simulink model "M10B39_es_V1"  (R2024b)
settings: Solver=ode23tb  StartTime=0.0  StopTime=20  FixedStep=0.001  RelTol=1e-3  EnableMultiTasking=on
InitFcn:
  | initAll;
values from neighbouring files (symbols this model uses):
  acom = 100    [initAll_V1.m]    (also in initAll_V2.m; initAll_V3.m; parameterinit.mat)
  AVm0 = [4.26082678503 4.656135219]    [parameterinit.mat]
  bcom = 50    [initAll_V1.m]    (also in initAll_V2.m; initAll_V3.m; parameterinit.mat)
  commun = 0*commun    [initAll_V1.m]    (also in initAll_V2.m; initAll_V3.m; parameterinit.mat = [0  0  0; 0  0  0; 0  0  0; 0  0  0])
  DataDelay = 0.0*DataDelay    [initAll_V1.m]    (also in initAll_V2.m; initAll_V3.m; parameterinit.mat = [0  0  0; 0  0  0; 0  0  0; 0  0  0])
  ESinit =     [parameterinit.mat]
  fB = 50    [initAll.m]    (also in initAll_V1.m; initAll_V2.m; initAll_V3.m; parameterinit.mat)
  Geninit = Generator_init(opdata,SynMach_in_gidx)    [initAll.m]    (also in initAll_V1.m; initAll_V2.m; initAll_V3.m = Generator_init(opdata_all,SynMach_in_gidx1); parameterinit.mat = )
  lam = 100    [initAll_V1.m]    (also in initAll_V2.m; initAll_V3.m; parameterinit.mat)
  SgridB = 100    [initAll.m]    (also in initAll_V1.m; initAll_V2.m; initAll_V3.m; parameterinit.mat)
  wB = 2*pi*fB    (= 314.159265359)    [initAll.m]    (also in initAll_V1.m; initAll_V2.m; initAll_V3.m; parameterinit.mat)
  Windinit =     [parameterinit.mat]
  YY_load = [3.65450097002 -2.05705688056 0 0 0 0 0 0 0 0 0 0 ... (1521 elements, 39x39)]    [parameterinit.mat]    (also in powerflowcaculate.m = full(YY))
undefined symbols (not defined in the file or in its folder): c1, c2, c3, c4, c5, c6, cp_nom, lambda_nom, P_wind_base, Pelec_base, Pnom
libraries: spsBistableLib x12, simulink_extras x4, slpidlib x1, simulink x1
(part 3 of 7)

== system M10B39_es_V1/Genrators/W_ES ==
  Gain1 : Gain  Gain=commun(4,1)
  Gain10 : Gain  Gain=commun(3,1)
  Gain11 : Gain  Gain=commun(1,2)
  Gain12 : Gain  Gain=commun(2,1)
  Gain13 : Gain  Gain=commun(8,2)
  Gain2 : Gain  Gain=commun(2,2)
  Gain26 : Gain  Gain=commun(8,1)
  Gain27 : Gain  Gain=commun(6,2)
  Gain28 : Gain  Gain=commun(1,1)
  Gain29 : Gain  Gain=commun(7,2)
  Gain3 : Gain  Gain=commun(5,1)
  Gain4 : Gain  Gain=commun(3,2)
  Gain5 : Gain  Gain=commun(6,1)
  Gain6 : Gain  Gain=commun(4,2)
  Gain7 : Gain  Gain=commun(7,1)
  Gain8 : Gain  Gain=commun(5,2)
  Mux : Mux
  Mux1 : Mux
  Mux{15..19,25,32..33} (8 alike) : Mux  Inputs=3
  Mux2 : Mux  Inputs=2
  Transport Delay1 : TransportDelay  DelayTime=DataDelay(4,1)
  Transport Delay10 : TransportDelay  DelayTime=DataDelay(5,2)
  Transport Delay16 : TransportDelay  DelayTime=DataDelay(2,1)
  Transport Delay17 : TransportDelay  DelayTime=DataDelay(8,2)
  Transport Delay2 : TransportDelay  DelayTime=DataDelay(1,2)
  Transport Delay25 : TransportDelay  DelayTime=DataDelay(7,2)
  Transport Delay26 : TransportDelay  DelayTime=DataDelay(8,1)
  Transport Delay27 : TransportDelay  DelayTime=DataDelay(6,2)
  Transport Delay28 : TransportDelay  DelayTime=DataDelay(1,1)
  Transport Delay3 : TransportDelay  DelayTime=DataDelay(3,1)
  Transport Delay4 : TransportDelay  DelayTime=DataDelay(2,2)
  Transport Delay5 : TransportDelay  DelayTime=DataDelay(5,1)
  Transport Delay6 : TransportDelay  DelayTime=DataDelay(3,2)
  Transport Delay7 : TransportDelay  DelayTime=DataDelay(6,1)
  Transport Delay8 : TransportDelay  DelayTime=DataDelay(4,2)
  Transport Delay9 : TransportDelay  DelayTime=DataDelay(7,1)
  W_ES : Outport
  wires:
  Gain26/1 -> Transport Delay26/1
  Transport Delay28/1 -> Mux33/1
  Gain5/1 -> Transport Delay7/1
  [WreES4] -> Gain6/1
  [WreES8] -> Gain26/1
  [WreES3] -> Gain10/1  "W3"
  [WreES6] -> Mux25/3
  Transport Delay8/1 -> Mux19/2
  Transport Delay2/1 -> Mux16/2
  [WreES1] -> Gain28/1
  [WreES7] -> Gain29/1
  Transport Delay25/1 -> Mux33/2
  [WreES6] -> Gain5/1
  [WreES1] -> Mux15/3  "W1"
  Gain11/1 -> Transport Delay2/1
  Transport Delay16/1 -> Mux15/1
  Transport Delay10/1 -> Mux25/2
  Gain3/1 -> Transport Delay5/1
  Transport Delay26/1 -> Mux32/1
  Mux32/1 -> Mux1/3  "W_ES7"
  Transport Delay3/1 -> Mux16/1
  [WreES8] -> Mux33/3
  Gain28/1 -> Transport Delay28/1
  Transport Delay5/1 -> Mux18/1
  Gain27/1 -> Transport Delay27/1
  Mux18/1 -> Mux/4  "W_ES4"
  Transport Delay9/1 -> Mux25/1
  [WreES2] -> Mux16/3  "W2"
  Gain6/1 -> Transport Delay8/1
  [WreES7] -> Mux32/3
  [WreES2] -> Gain2/1  "W2"
  Transport Delay1/1 -> Mux17/1
  [WreES1] -> Gain11/1  "W1"
  Gain10/1 -> Transport Delay3/1
  Gain4/1 -> Transport Delay6/1
  Transport Delay6/1 -> Mux18/2
  Mux25/1 -> Mux1/2  "W_ES6"
  Mux15/1 -> Mux/1  "W_ES1"
  Gain1/1 -> Transport Delay1/1
  Gain13/1 -> Transport Delay17/1
  [WreES4] -> Gain1/1  "W4"
  [WreES3] -> Mux17/3  "W3"
  Transport Delay7/1 -> Mux19/1
  Transport Delay4/1 -> Mux17/2
  [WreES5] -> Mux19/3
  Gain29/1 -> Transport Delay25/1
  [WreES4] -> Mux18/3  "W4"
  Transport Delay17/1 -> Mux15/2
  Gain12/1 -> Transport Delay16/1
  Transport Delay27/1 -> Mux32/2
  [WreES5] -> Gain3/1
  [WreES2] -> Gain12/1  "W2"
  [WreES8] -> Gain13/1  "W4"
  Mux33/1 -> Mux1/4  "W_ES8"
  [WreES6] -> Gain27/1
  Gain7/1 -> Transport Delay9/1
  Gain2/1 -> Transport Delay4/1
  Gain8/1 -> Transport Delay10/1
  Mux17/1 -> Mux/3  "W_ES3"
  [WreES7] -> Gain7/1
  [WreES5] -> Gain8/1
  Mux16/1 -> Mux/2  "W_ES2"
  [WreES3] -> Gain4/1  "W3"
  Mux19/1 -> Mux1/1  "W_ES5"
  Mux/1 -> Mux2/1
  Mux1/1 -> Mux2/2
  Mux2/1 -> W_ES/1

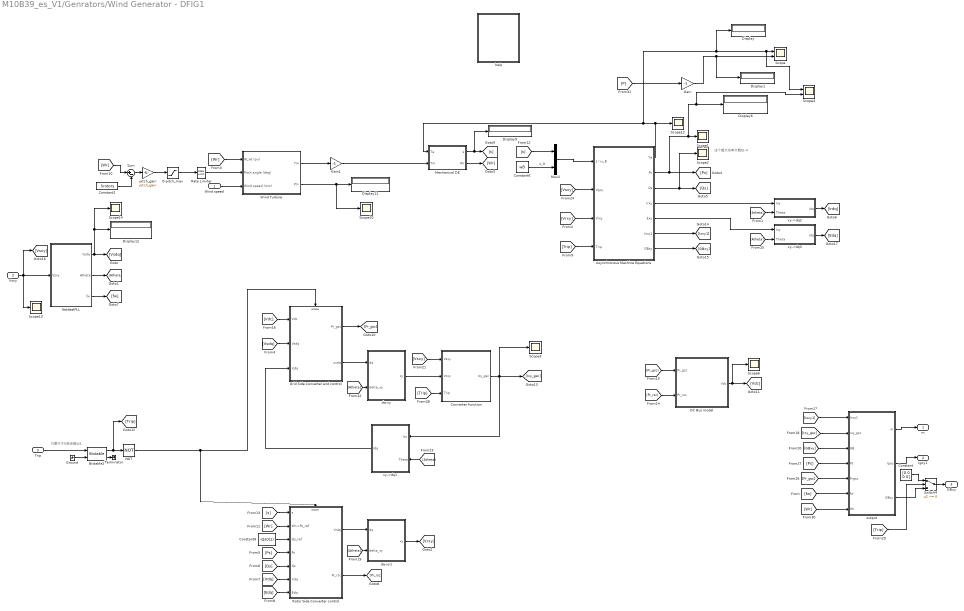
== system M10B39_es_V1/Genrators/Wind Generator - DFIG1 ==
  note: 只要大于0就会输出1
  note: 这个最大功率大概在-4
  Wind speed : Inport
  Vsxy : Inport  Port=2
  Trip : Inport  Port=3
  0-pitch_max : Saturate  UpperLimit=pitch_max  LowerLimit=0
  "Asynchronous Machine Equations " : Subsystem
  Bistable2 : spsBistableLib/Bistable  Qpriority=Set  ic=0  Ts=0
  Constant : Constant  Value=[0 0 0 0]
  Constant2 : Constant  Value=Srotors
  Constant6 : Constant  Value=wB
  Constant8 : Constant  Value=-Qs0(1)
  Converter function : Subsystem
  DC Bus model : Subsystem
  Display{,1,6,9,11..12} (6 alike) : Display
  Gain : Gain  Gain=-1
  Gain1 : Gain  Gain=-1
  Grid Side Converter and control : Subsystem
  Ground : Ground
  Mechanical DE : Subsystem
  Mux2 : Mux  Inputs=2
  NOT : Logic  Operator=NOT  AllPortsSameDT=off  OutDataTypeStr=boolean
  NoIdealPLL : Subsystem  VariantControl=Noideal_PLL_Wind1
  "Rate Limiter   " : RateLimiter  RisingSlewLimit=pitch_rate  FallingSlewLimit=-pitch_rate
  Rotor Side Converter control : Subsystem
  Scope : Scope  NumInputPorts=2
  Scope{1..3,6,10,12..14} (8 alike) : Scope
  Scope4 : Scope  NumInputPorts=2
  Sum : Sum  Inputs=|+-  SaturateOnIntegerOverflow=on
  Switch4 : Switch  Criteria=u2 ~= 0  Threshold=0.5  InputSameDT=off
  Terminator : Terminator
  Wind Turbine : Subsystem
  dq-xy : Subsystem
  dq-xy1 : Subsystem
  help : Subsystem
  output : Subsystem
  pitch_gain : Gain  Gain=pitch_gain  SaturateOnIntegerOverflow=on  OutDataTypeStr=Inherit: Same as input  ParamDataTypeStr=Inherit: Same as input
  xy->dq1 : Subsystem
  xy->dq2 : Subsystem
  xy->dq3 : Subsystem
  m : Outport
  Igxy1 : Outport  Port=2
  GBxy : Outport  Port=3
  wires:
  [Wr] -> output/7(Wr)
  Gain1/1 -> Mechanical DE/2(Tm)
  output/3(GBxy) -> Switch4/3
  Switch4/1 -> GBxy/1
  Constant/1 -> Switch4/1
  [Trip] -> Switch4/2
  [Trip] -> Converter function/3(Trip)
  [Trip] -> "Asynchronous Machine Equations "/4("Trip ")
  [Wr] -> Sum/1
  0-pitch_max/1 -> "Rate Limiter   "/1
  pitch_gain/1 -> 0-pitch_max/1
  Constant2/1 -> Sum/2
  Sum/1 -> pitch_gain/1
  NOT/1 -> Rotor Side Converter control/Enable, Grid Side Converter and control/Enable
  Trip/1 -> Bistable2/1
  Bistable2/2 -> Terminator/1
  Bistable2/1 -> NOT/1, [Trip]
  Ground/1 -> Bistable2/2
  [fw] -> output/6(fw)
  [Pr_gsc] -> output/5(Prgsc)
  [Ps] -> output/4(Ps)
  output/1(m) -> m/1
  [Isxy1] -> output/1(Isxy1)
  [Ixy_gsc] -> output/2(Ixy_gsc)
  output/2(Igxy) -> Igxy1/1
  xy->dq3/1(Idq) -> [Edq]
  [Atheta] -> xy->dq3/2(Theta)
  xy->dq2/1(Idq) -> [Irdq]
  [Atheta] -> xy->dq2/2(Theta)
  dq-xy1/1(xy) -> [Vrxy]
  [Atheta] -> dq-xy1/2(delta_xy)
  xy->dq1/1(Idq) -> Grid Side Converter and control/3(Icdq)
  [Atheta] -> xy->dq1/2(Theta)
  [Atheta] -> dq-xy/2(delta_xy)
  dq-xy/1(xy) -> Converter function/2(Vcxy)
  Grid Side Converter and control/2(ucdq) -> dq-xy/1(dq)
  [Vsxy] -> Converter function/1(Vsxy)
  NoIdealPLL/3(fw) -> [fw]
  Vsxy/1 -> [Vsxy], Scope13/1, NoIdealPLL/1(Vsxy)
  [GBxy] -> output/3(GB)
  [Pr_rsc] -> DC Bus model/2(Pr_rsc)
  "Asynchronous Machine Equations "/1(Te) -> Scope12/1, Display/1, Scope4/1, Scope/1, Mechanical DE/1(Te)
  Constant8/1 -> Rotor Side Converter control/3(Qs_ref)
  [Wr] -> Wind Turbine/1(W_wt (pu))
  "Asynchronous Machine Equations "/4(Irxy) -> xy->dq2/1(Ixy)
  Converter function/1(Ixy_gsc) -> [Ixy_gsc], xy->dq1/1(Ixy), Scope3/1
  [Vrxy] -> "Asynchronous Machine Equations "/3(Vrxy)
  "Asynchronous Machine Equations "/6(Isxy1) -> [Isxy1]
  [Qs] -> Rotor Side Converter control/5(Qs)
  [Vdc] -> Grid Side Converter and control/1(Vdc)
  [Pr_gsc] -> DC Bus model/1(Pr_gsc)
  "Asynchronous Machine Equations "/2(Ps) -> Scope1/1, Scope4/2, Display6/1, [Ps]
  Mechanical DE/1("s ") -> [s], Display9/1
  [s] -> Mux2/1
  [Vsdq] -> Grid Side Converter and control/2(Vsdq)
  Grid Side Converter and control/1(Pr_gsc) -> [Pr_gsc]
  NoIdealPLL/2(Atheta) -> [Atheta]
  DC Bus model/1(Vdc) -> [Vdc], Scope6/1
  [Vsxy] -> "Asynchronous Machine Equations "/2(Vgxy)
  Wind Turbine/1(Tm) -> Gain1/1
  [Irdq] -> Rotor Side Converter control/6(Irdq)
  Mux2/1 -> "Asynchronous Machine Equations "/1(s / ω_B)
  "Asynchronous Machine Equations "/7(GBxy) -> [GBxy]
  "Rate Limiter   "/1 -> Wind Turbine/2(Pitch angle (deg))
  NoIdealPLL/1(Vsdq) -> Display12/1, Scope14/1, [Vsdq]
  [s] -> Rotor Side Converter control/1(s)
  Rotor Side Converter control/2(Pr_rsc) -> [Pr_rsc]
  Mechanical DE/2(Wr) -> [Wr]
  [Wr] -> Rotor Side Converter control/2(Wr->Ps_ref)
  Wind Turbine/2(Pm) -> Display11/1, Scope10/1
  "Asynchronous Machine Equations "/3(Qs) -> [Qs], Scope2/1
  Wind speed/1 -> Wind Turbine/3(Wind speed (m/s))
  [Ps] -> Rotor Side Converter control/4(Ps)
  Rotor Side Converter control/1(Vrdq) -> dq-xy1/1(dq)
  [Edq] -> Rotor Side Converter control/7(Edq)
  Constant6/1 -> Mux2/2  "w_B"
  "Asynchronous Machine Equations "/5(Exy) -> xy->dq3/1(Ixy)
  [P] -> Gain/1
  Gain/1 -> Display1/1, Scope/2

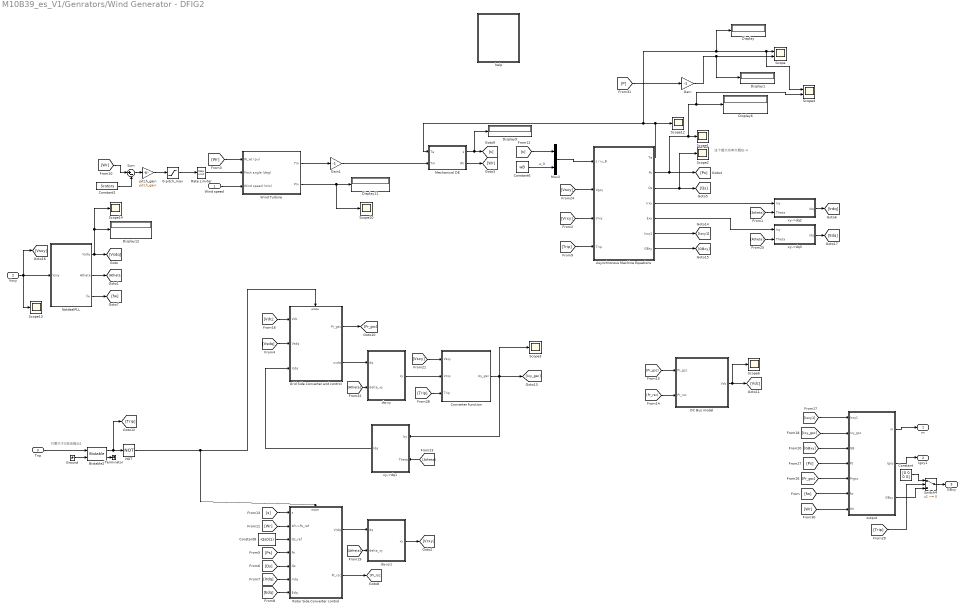
== system M10B39_es_V1/Genrators/Wind Generator - DFIG2 ==
  note: 只要大于0就会输出1
  note: 这个最大功率大概在-4
  Wind speed : Inport
  Vsxy : Inport  Port=2
  Trip : Inport  Port=3
  0-pitch_max : Saturate  UpperLimit=pitch_max  LowerLimit=0
  "Asynchronous Machine Equations " : Subsystem
  Bistable2 : spsBistableLib/Bistable  Qpriority=Set  ic=0  Ts=0
  Constant : Constant  Value=[0 0 0 0]
  Constant2 : Constant  Value=Srotors
  Constant6 : Constant  Value=wB
  Constant8 : Constant  Value=-Qs0(1)
  Converter function : Subsystem
  DC Bus model : Subsystem
  Display{,1,6,9,11..12} (6 alike) : Display
  Gain : Gain  Gain=-1
  Gain1 : Gain  Gain=-1
  Grid Side Converter and control : Subsystem
  Ground : Ground
  Mechanical DE : Subsystem
  Mux2 : Mux  Inputs=2
  NOT : Logic  Operator=NOT  AllPortsSameDT=off  OutDataTypeStr=boolean
  NoIdealPLL : Subsystem  VariantControl=Noideal_PLL_Wind1
  "Rate Limiter   " : RateLimiter  RisingSlewLimit=pitch_rate  FallingSlewLimit=-pitch_rate
  Rotor Side Converter control : Subsystem
  Scope : Scope  NumInputPorts=2
  Scope{1..3,6,10,12..14} (8 alike) : Scope
  Scope4 : Scope  NumInputPorts=2
  Sum : Sum  Inputs=|+-  SaturateOnIntegerOverflow=on
  Switch4 : Switch  Criteria=u2 ~= 0  Threshold=0.5  InputSameDT=off
  Terminator : Terminator
  Wind Turbine : Subsystem
  dq-xy : Subsystem
  dq-xy1 : Subsystem
  help : Subsystem
  output : Subsystem
  pitch_gain : Gain  Gain=pitch_gain  SaturateOnIntegerOverflow=on  OutDataTypeStr=Inherit: Same as input  ParamDataTypeStr=Inherit: Same as input
  xy->dq1 : Subsystem
  xy->dq2 : Subsystem
  xy->dq3 : Subsystem
  m : Outport
  Igxy1 : Outport  Port=2
  GBxy : Outport  Port=3
  wires:
  [Wr] -> output/7(Wr)
  Gain1/1 -> Mechanical DE/2(Tm)
  output/3(GBxy) -> Switch4/3
  Switch4/1 -> GBxy/1
  Constant/1 -> Switch4/1
  [Trip] -> Switch4/2
  [Trip] -> Converter function/3(Trip)
  [Trip] -> "Asynchronous Machine Equations "/4("Trip ")
  [Wr] -> Sum/1
  0-pitch_max/1 -> "Rate Limiter   "/1
  pitch_gain/1 -> 0-pitch_max/1
  Constant2/1 -> Sum/2
  Sum/1 -> pitch_gain/1
  NOT/1 -> Rotor Side Converter control/Enable, Grid Side Converter and control/Enable
  Trip/1 -> Bistable2/1
  Bistable2/2 -> Terminator/1
  Bistable2/1 -> NOT/1, [Trip]
  Ground/1 -> Bistable2/2
  [fw] -> output/6(fw)
  [Pr_gsc] -> output/5(Prgsc)
  [Ps] -> output/4(Ps)
  output/1(m) -> m/1
  [Isxy1] -> output/1(Isxy1)
  [Ixy_gsc] -> output/2(Ixy_gsc)
  output/2(Igxy) -> Igxy1/1
  xy->dq3/1(Idq) -> [Edq]
  [Atheta] -> xy->dq3/2(Theta)
  xy->dq2/1(Idq) -> [Irdq]
  [Atheta] -> xy->dq2/2(Theta)
  dq-xy1/1(xy) -> [Vrxy]
  [Atheta] -> dq-xy1/2(delta_xy)
  xy->dq1/1(Idq) -> Grid Side Converter and control/3(Icdq)
  [Atheta] -> xy->dq1/2(Theta)
  [Atheta] -> dq-xy/2(delta_xy)
  dq-xy/1(xy) -> Converter function/2(Vcxy)
  Grid Side Converter and control/2(ucdq) -> dq-xy/1(dq)
  [Vsxy] -> Converter function/1(Vsxy)
  NoIdealPLL/3(fw) -> [fw]
  Vsxy/1 -> [Vsxy], Scope13/1, NoIdealPLL/1(Vsxy)
  [GBxy] -> output/3(GB)
  [Pr_rsc] -> DC Bus model/2(Pr_rsc)
  "Asynchronous Machine Equations "/1(Te) -> Scope12/1, Display/1, Scope4/1, Scope/1, Mechanical DE/1(Te)
  Constant8/1 -> Rotor Side Converter control/3(Qs_ref)
  [Wr] -> Wind Turbine/1(W_wt (pu))
  "Asynchronous Machine Equations "/4(Irxy) -> xy->dq2/1(Ixy)
  Converter function/1(Ixy_gsc) -> [Ixy_gsc], xy->dq1/1(Ixy), Scope3/1
  [Vrxy] -> "Asynchronous Machine Equations "/3(Vrxy)
  "Asynchronous Machine Equations "/6(Isxy1) -> [Isxy1]
  [Qs] -> Rotor Side Converter control/5(Qs)
  [Vdc] -> Grid Side Converter and control/1(Vdc)
  [Pr_gsc] -> DC Bus model/1(Pr_gsc)
  "Asynchronous Machine Equations "/2(Ps) -> Scope1/1, Scope4/2, Display6/1, [Ps]
  Mechanical DE/1("s ") -> [s], Display9/1
  [s] -> Mux2/1
  [Vsdq] -> Grid Side Converter and control/2(Vsdq)
  Grid Side Converter and control/1(Pr_gsc) -> [Pr_gsc]
  NoIdealPLL/2(Atheta) -> [Atheta]
  DC Bus model/1(Vdc) -> [Vdc], Scope6/1
  [Vsxy] -> "Asynchronous Machine Equations "/2(Vgxy)
  Wind Turbine/1(Tm) -> Gain1/1
  [Irdq] -> Rotor Side Converter control/6(Irdq)
  Mux2/1 -> "Asynchronous Machine Equations "/1(s / ω_B)
  "Asynchronous Machine Equations "/7(GBxy) -> [GBxy]
  "Rate Limiter   "/1 -> Wind Turbine/2(Pitch angle (deg))
  NoIdealPLL/1(Vsdq) -> Display12/1, Scope14/1, [Vsdq]
  [s] -> Rotor Side Converter control/1(s)
  Rotor Side Converter control/2(Pr_rsc) -> [Pr_rsc]
  Mechanical DE/2(Wr) -> [Wr]
  [Wr] -> Rotor Side Converter control/2(Wr->Ps_ref)
  Wind Turbine/2(Pm) -> Display11/1, Scope10/1
  "Asynchronous Machine Equations "/3(Qs) -> [Qs], Scope2/1
  Wind speed/1 -> Wind Turbine/3(Wind speed (m/s))
  [Ps] -> Rotor Side Converter control/4(Ps)
  Rotor Side Converter control/1(Vrdq) -> dq-xy1/1(dq)
  [Edq] -> Rotor Side Converter control/7(Edq)
  Constant6/1 -> Mux2/2  "w_B"
  "Asynchronous Machine Equations "/5(Exy) -> xy->dq3/1(Ixy)
  [P] -> Gain/1
  Gain/1 -> Display1/1, Scope/2

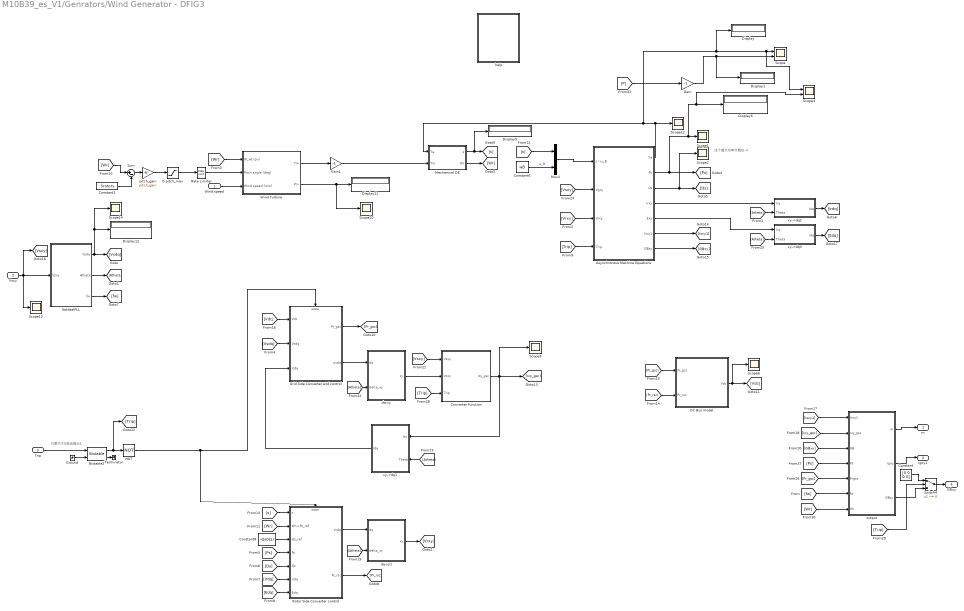
== system M10B39_es_V1/Genrators/Wind Generator - DFIG3 ==
  note: 只要大于0就会输出1
  note: 这个最大功率大概在-4
  Wind speed : Inport
  Vsxy : Inport  Port=2
  Trip : Inport  Port=3
  0-pitch_max : Saturate  UpperLimit=pitch_max  LowerLimit=0
  "Asynchronous Machine Equations " : Subsystem
  Bistable2 : spsBistableLib/Bistable  Qpriority=Set  ic=0  Ts=0
  Constant : Constant  Value=[0 0 0 0]
  Constant2 : Constant  Value=Srotors
  Constant6 : Constant  Value=wB
  Constant8 : Constant  Value=-Qs0(1)
  Converter function : Subsystem
  DC Bus model : Subsystem
  Display{,1,6,9,11..12} (6 alike) : Display
  Gain : Gain  Gain=-1
  Gain1 : Gain  Gain=-1
  Grid Side Converter and control : Subsystem
  Ground : Ground
  Mechanical DE : Subsystem
  Mux2 : Mux  Inputs=2
  NOT : Logic  Operator=NOT  AllPortsSameDT=off  OutDataTypeStr=boolean
  NoIdealPLL : Subsystem  VariantControl=Noideal_PLL_Wind1
  "Rate Limiter   " : RateLimiter  RisingSlewLimit=pitch_rate  FallingSlewLimit=-pitch_rate
  Rotor Side Converter control : Subsystem
  Scope : Scope  NumInputPorts=2
  Scope{1..3,6,10,12..14} (8 alike) : Scope
  Scope4 : Scope  NumInputPorts=2
  Sum : Sum  Inputs=|+-  SaturateOnIntegerOverflow=on
  Switch4 : Switch  Criteria=u2 ~= 0  Threshold=0.5  InputSameDT=off
  Terminator : Terminator
  Wind Turbine : Subsystem
  dq-xy : Subsystem
  dq-xy1 : Subsystem
  help : Subsystem
  output : Subsystem
  pitch_gain : Gain  Gain=pitch_gain  SaturateOnIntegerOverflow=on  OutDataTypeStr=Inherit: Same as input  ParamDataTypeStr=Inherit: Same as input
  xy->dq1 : Subsystem
  xy->dq2 : Subsystem
  xy->dq3 : Subsystem
  m : Outport
  Igxy1 : Outport  Port=2
  GBxy : Outport  Port=3
  wires:
  [Wr] -> output/7(Wr)
  Gain1/1 -> Mechanical DE/2(Tm)
  output/3(GBxy) -> Switch4/3
  Switch4/1 -> GBxy/1
  Constant/1 -> Switch4/1
  [Trip] -> Switch4/2
  [Trip] -> Converter function/3(Trip)
  [Trip] -> "Asynchronous Machine Equations "/4("Trip ")
  [Wr] -> Sum/1
  0-pitch_max/1 -> "Rate Limiter   "/1
  pitch_gain/1 -> 0-pitch_max/1
  Constant2/1 -> Sum/2
  Sum/1 -> pitch_gain/1
  NOT/1 -> Rotor Side Converter control/Enable, Grid Side Converter and control/Enable
  Trip/1 -> Bistable2/1
  Bistable2/2 -> Terminator/1
  Bistable2/1 -> NOT/1, [Trip]
  Ground/1 -> Bistable2/2
  [fw] -> output/6(fw)
  [Pr_gsc] -> output/5(Prgsc)
  [Ps] -> output/4(Ps)
  output/1(m) -> m/1
  [Isxy1] -> output/1(Isxy1)
  [Ixy_gsc] -> output/2(Ixy_gsc)
  output/2(Igxy) -> Igxy1/1
  xy->dq3/1(Idq) -> [Edq]
  [Atheta] -> xy->dq3/2(Theta)
  xy->dq2/1(Idq) -> [Irdq]
  [Atheta] -> xy->dq2/2(Theta)
  dq-xy1/1(xy) -> [Vrxy]
  [Atheta] -> dq-xy1/2(delta_xy)
  xy->dq1/1(Idq) -> Grid Side Converter and control/3(Icdq)
  [Atheta] -> xy->dq1/2(Theta)
  [Atheta] -> dq-xy/2(delta_xy)
  dq-xy/1(xy) -> Converter function/2(Vcxy)
  Grid Side Converter and control/2(ucdq) -> dq-xy/1(dq)
  [Vsxy] -> Converter function/1(Vsxy)
  NoIdealPLL/3(fw) -> [fw]
  Vsxy/1 -> [Vsxy], Scope13/1, NoIdealPLL/1(Vsxy)
  [GBxy] -> output/3(GB)
  [Pr_rsc] -> DC Bus model/2(Pr_rsc)
  "Asynchronous Machine Equations "/1(Te) -> Scope12/1, Display/1, Scope4/1, Scope/1, Mechanical DE/1(Te)
  Constant8/1 -> Rotor Side Converter control/3(Qs_ref)
  [Wr] -> Wind Turbine/1(W_wt (pu))
  "Asynchronous Machine Equations "/4(Irxy) -> xy->dq2/1(Ixy)
  Converter function/1(Ixy_gsc) -> [Ixy_gsc], xy->dq1/1(Ixy), Scope3/1
  [Vrxy] -> "Asynchronous Machine Equations "/3(Vrxy)
  "Asynchronous Machine Equations "/6(Isxy1) -> [Isxy1]
  [Qs] -> Rotor Side Converter control/5(Qs)
  [Vdc] -> Grid Side Converter and control/1(Vdc)
  [Pr_gsc] -> DC Bus model/1(Pr_gsc)
  "Asynchronous Machine Equations "/2(Ps) -> Scope1/1, Scope4/2, Display6/1, [Ps]
  Mechanical DE/1("s ") -> [s], Display9/1
  [s] -> Mux2/1
  [Vsdq] -> Grid Side Converter and control/2(Vsdq)
  Grid Side Converter and control/1(Pr_gsc) -> [Pr_gsc]
  NoIdealPLL/2(Atheta) -> [Atheta]
  DC Bus model/1(Vdc) -> [Vdc], Scope6/1
  [Vsxy] -> "Asynchronous Machine Equations "/2(Vgxy)
  Wind Turbine/1(Tm) -> Gain1/1
  [Irdq] -> Rotor Side Converter control/6(Irdq)
  Mux2/1 -> "Asynchronous Machine Equations "/1(s / ω_B)
  "Asynchronous Machine Equations "/7(GBxy) -> [GBxy]
  "Rate Limiter   "/1 -> Wind Turbine/2(Pitch angle (deg))
  NoIdealPLL/1(Vsdq) -> Display12/1, Scope14/1, [Vsdq]
  [s] -> Rotor Side Converter control/1(s)
  Rotor Side Converter control/2(Pr_rsc) -> [Pr_rsc]
  Mechanical DE/2(Wr) -> [Wr]
  [Wr] -> Rotor Side Converter control/2(Wr->Ps_ref)
  Wind Turbine/2(Pm) -> Display11/1, Scope10/1
  "Asynchronous Machine Equations "/3(Qs) -> [Qs], Scope2/1
  Wind speed/1 -> Wind Turbine/3(Wind speed (m/s))
  [Ps] -> Rotor Side Converter control/4(Ps)
  Rotor Side Converter control/1(Vrdq) -> dq-xy1/1(dq)
  [Edq] -> Rotor Side Converter control/7(Edq)
  Constant6/1 -> Mux2/2  "w_B"
  "Asynchronous Machine Equations "/5(Exy) -> xy->dq3/1(Ixy)
  [P] -> Gain/1
  Gain/1 -> Display1/1, Scope/2

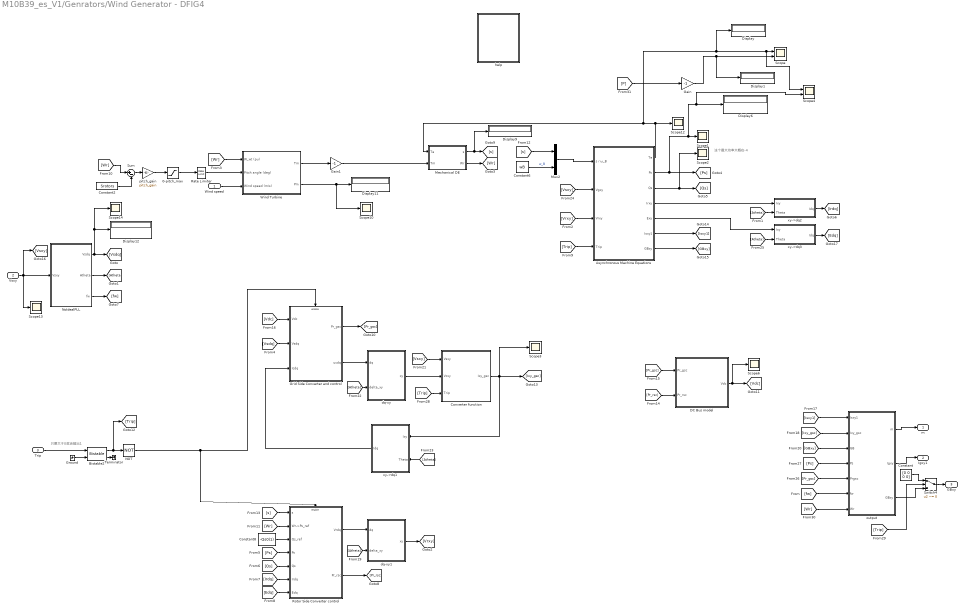
== system M10B39_es_V1/Genrators/Wind Generator - DFIG4 ==
  note: 只要大于0就会输出1
  note: 这个最大功率大概在-4
  Wind speed : Inport
  Vsxy : Inport  Port=2
  Trip : Inport  Port=3
  0-pitch_max : Saturate  UpperLimit=pitch_max  LowerLimit=0
  "Asynchronous Machine Equations " : Subsystem
  Bistable2 : spsBistableLib/Bistable  Qpriority=Set  ic=0  Ts=0
  Constant : Constant  Value=[0 0 0 0]
  Constant2 : Constant  Value=Srotors
  Constant6 : Constant  Value=wB
  Constant8 : Constant  Value=-Qs0(1)
  Converter function : Subsystem
  DC Bus model : Subsystem
  Display{,1,6,9,11..12} (6 alike) : Display
  Gain : Gain  Gain=-1
  Gain1 : Gain  Gain=-1
  Grid Side Converter and control : Subsystem
  Ground : Ground
  Mechanical DE : Subsystem
  Mux2 : Mux  Inputs=2
  NOT : Logic  Operator=NOT  AllPortsSameDT=off  OutDataTypeStr=boolean
  NoIdealPLL : Subsystem  VariantControl=Noideal_PLL_Wind1
  "Rate Limiter   " : RateLimiter  RisingSlewLimit=pitch_rate  FallingSlewLimit=-pitch_rate
  Rotor Side Converter control : Subsystem
  Scope : Scope  NumInputPorts=2
  Scope{1..3,6,10,12..14} (8 alike) : Scope
  Scope4 : Scope  NumInputPorts=2
  Sum : Sum  Inputs=|+-  SaturateOnIntegerOverflow=on
  Switch4 : Switch  Criteria=u2 ~= 0  Threshold=0.5  InputSameDT=off
  Terminator : Terminator
  Wind Turbine : Subsystem
  dq-xy : Subsystem
  dq-xy1 : Subsystem
  help : Subsystem
  output : Subsystem
  pitch_gain : Gain  Gain=pitch_gain  SaturateOnIntegerOverflow=on  OutDataTypeStr=Inherit: Same as input  ParamDataTypeStr=Inherit: Same as input
  xy->dq1 : Subsystem
  xy->dq2 : Subsystem
  xy->dq3 : Subsystem
  m : Outport
  Igxy1 : Outport  Port=2
  GBxy : Outport  Port=3
  wires:
  [Wr] -> output/7(Wr)
  Gain1/1 -> Mechanical DE/2(Tm)
  output/3(GBxy) -> Switch4/3
  Switch4/1 -> GBxy/1
  Constant/1 -> Switch4/1
  [Trip] -> Switch4/2
  [Trip] -> Converter function/3(Trip)
  [Trip] -> "Asynchronous Machine Equations "/4("Trip ")
  [Wr] -> Sum/1
  0-pitch_max/1 -> "Rate Limiter   "/1
  pitch_gain/1 -> 0-pitch_max/1
  Constant2/1 -> Sum/2
  Sum/1 -> pitch_gain/1
  NOT/1 -> Rotor Side Converter control/Enable, Grid Side Converter and control/Enable
  Trip/1 -> Bistable2/1
  Bistable2/2 -> Terminator/1
  Bistable2/1 -> NOT/1, [Trip]
  Ground/1 -> Bistable2/2
  [fw] -> output/6(fw)
  [Pr_gsc] -> output/5(Prgsc)
  [Ps] -> output/4(Ps)
  output/1(m) -> m/1
  [Isxy1] -> output/1(Isxy1)
  [Ixy_gsc] -> output/2(Ixy_gsc)
  output/2(Igxy) -> Igxy1/1
  xy->dq3/1(Idq) -> [Edq]
  [Atheta] -> xy->dq3/2(Theta)
  xy->dq2/1(Idq) -> [Irdq]
  [Atheta] -> xy->dq2/2(Theta)
  dq-xy1/1(xy) -> [Vrxy]
  [Atheta] -> dq-xy1/2(delta_xy)
  xy->dq1/1(Idq) -> Grid Side Converter and control/3(Icdq)
  [Atheta] -> xy->dq1/2(Theta)
  [Atheta] -> dq-xy/2(delta_xy)
  dq-xy/1(xy) -> Converter function/2(Vcxy)
  Grid Side Converter and control/2(ucdq) -> dq-xy/1(dq)
  [Vsxy] -> Converter function/1(Vsxy)
  NoIdealPLL/3(fw) -> [fw]
  Vsxy/1 -> [Vsxy], Scope13/1, NoIdealPLL/1(Vsxy)
  [GBxy] -> output/3(GB)
  [Pr_rsc] -> DC Bus model/2(Pr_rsc)
  "Asynchronous Machine Equations "/1(Te) -> Scope12/1, Display/1, Scope4/1, Scope/1, Mechanical DE/1(Te)
  Constant8/1 -> Rotor Side Converter control/3(Qs_ref)
  [Wr] -> Wind Turbine/1(W_wt (pu))
  "Asynchronous Machine Equations "/4(Irxy) -> xy->dq2/1(Ixy)
  Converter function/1(Ixy_gsc) -> [Ixy_gsc], xy->dq1/1(Ixy), Scope3/1
  [Vrxy] -> "Asynchronous Machine Equations "/3(Vrxy)
  "Asynchronous Machine Equations "/6(Isxy1) -> [Isxy1]
  [Qs] -> Rotor Side Converter control/5(Qs)
  [Vdc] -> Grid Side Converter and control/1(Vdc)
  [Pr_gsc] -> DC Bus model/1(Pr_gsc)
  "Asynchronous Machine Equations "/2(Ps) -> Scope1/1, Scope4/2, Display6/1, [Ps]
  Mechanical DE/1("s ") -> [s], Display9/1
  [s] -> Mux2/1
  [Vsdq] -> Grid Side Converter and control/2(Vsdq)
  Grid Side Converter and control/1(Pr_gsc) -> [Pr_gsc]
  NoIdealPLL/2(Atheta) -> [Atheta]
  DC Bus model/1(Vdc) -> [Vdc], Scope6/1
  [Vsxy] -> "Asynchronous Machine Equations "/2(Vgxy)
  Wind Turbine/1(Tm) -> Gain1/1
  [Irdq] -> Rotor Side Converter control/6(Irdq)
  Mux2/1 -> "Asynchronous Machine Equations "/1(s / ω_B)
  "Asynchronous Machine Equations "/7(GBxy) -> [GBxy]
  "Rate Limiter   "/1 -> Wind Turbine/2(Pitch angle (deg))
  NoIdealPLL/1(Vsdq) -> Display12/1, Scope14/1, [Vsdq]
  [s] -> Rotor Side Converter control/1(s)
  Rotor Side Converter control/2(Pr_rsc) -> [Pr_rsc]
  Mechanical DE/2(Wr) -> [Wr]
  [Wr] -> Rotor Side Converter control/2(Wr->Ps_ref)
  Wind Turbine/2(Pm) -> Display11/1, Scope10/1
  "Asynchronous Machine Equations "/3(Qs) -> [Qs], Scope2/1
  Wind speed/1 -> Wind Turbine/3(Wind speed (m/s))
  [Ps] -> Rotor Side Converter control/4(Ps)
  Rotor Side Converter control/1(Vrdq) -> dq-xy1/1(dq)
  [Edq] -> Rotor Side Converter control/7(Edq)
  Constant6/1 -> Mux2/2  "w_B"
  "Asynchronous Machine Equations "/5(Exy) -> xy->dq3/1(Ixy)
  [P] -> Gain/1
  Gain/1 -> Display1/1, Scope/2

== system M10B39_es_V1/Genrators/ES1/ control1 ==
  usdq : Inport
  isdq : Inport  Port=2
  delta : Inport  Port=3
  Enable : EnablePort
  Add : Sum  Inputs=|-+
  Add2 : Sum  Inputs=|-+
  Add3 : Sum
  Add4 : Sum  Inputs=-+
  Add6 : Sum  Inputs=|++
  Add7 : Sum  Inputs=+-
  Complex to Magnitude-Angle : ComplexToMagnitudeAngle
  Complex to Real-Imag1 : ComplexToRealImag
  Constant : Constant
  Constant1 : Constant  Value=usd0
  Constant2 : Constant  Value=0
  Constant3 : Constant  Value=Q0
  Constant4 : Constant
  Demux : Demux  Outputs=2
  Demux1 : Demux  Outputs=2
  Gain : Gain  Gain=0.01
  Gain1 : Gain  Gain=-1
  K5 : Gain  Gain=Lpr  SaturateOnIntegerOverflow=on  OutDataTypeStr=Inherit: Same as input  ParamDataTypeStr=Inherit: Same as input
  K6 : Gain  Gain=Lpr  SaturateOnIntegerOverflow=on  OutDataTypeStr=Inherit: Same as input  ParamDataTypeStr=Inherit: Same as input
  Magnitude-Angle to Complex : MagnitudeAngleToComplex
  Product{1,4..6} (4 alike) : Product  RndMeth=Zero
  Real-Imag to Complex : RealImagToComplex
  Scope : Scope
  Scope1 : Scope
  Scope2 : Scope  NumInputPorts=2
  Scope3 : Scope  NumInputPorts=2
  Scope7 : Scope  NumInputPorts=2
  Sum : Sum  Inputs=|+-
  Sum2 : Sum  Inputs=|+-  SaturateOnIntegerOverflow=on
  Sum23 : Sum  Inputs=|+-  SaturateOnIntegerOverflow=on
  Sum9 : Sum  Inputs=|+-  SaturateOnIntegerOverflow=on
  control_AC_voltage : Subsystem  VariantControl=VSC1q_Variant2
  control_AC_voltage1 : Subsystem  VariantControl=VSC1q_Variant2
  in_D_PI : Subsystem  mask{KP_=KpId_VSC_A, KI_=KiId_VSC_A, Upper_limit=inf, Lower_limit=-inf, Upper_saturation_limit=inf, Lower_saturation_limit=-inf, integrator_init=Md_A_0}
      mask prompts: KP_ "比例系数P"; KI_ "积分系数I"; Upper_limit "限幅上限"; Lower_limit "限幅下限"; Upper_saturation_limit "积分饱和上限"; Lower_saturation_limit "积分饱和下限"; integrator_init "积分初始值"
      mask DialogControl Container4 Prompt: 控制参数
      mask DialogControl Container5 Prompt: 初始值
      mask Display: disp('PI')
  in_Q_PI : Subsystem  mask{KP_=KpIq_VSC_A, KI_=KiIq_VSC_A, Upper_limit=inf, Lower_limit=-inf, Upper_saturation_limit=inf, Lower_saturation_limit=-inf, integrator_init=Mq_A_0}
      mask prompts: KP_ "比例系数P"; KI_ "积分系数I"; Upper_limit "限幅上限"; Lower_limit "限幅下限"; Upper_saturation_limit "积分饱和上限"; Lower_saturation_limit "积分饱和下限"; integrator_init "积分初始值"
      mask DialogControl Container4 Prompt: 控制参数
      mask DialogControl Container5 Prompt: 初始值
      mask Display: disp('PI')
  ucx : Outport
  ucy : Outport  Port=2
  wires:
  Magnitude-Angle to Complex/1 -> Complex to Real-Imag1/1
  Add/1 -> Real-Imag to Complex/2
  Add2/1 -> Real-Imag to Complex/1
  delta/1 -> Add6/2
  Add6/1 -> Magnitude-Angle to Complex/2
  Complex to Magnitude-Angle/2 -> Add6/1
  Sum9/1 -> in_D_PI/1(In1)
  K5/1 -> Add3/1
  [usd] -> Add3/2
  Add3/1 -> Add2/2
  in_D_PI/1(Out1) -> Add2/1
  Constant/1 -> Product4/2
  [isq] -> Product4/1
  [isd] -> Scope7/2, Sum9/2
  Product4/1 -> K5/1
  Demux1/1 -> [isd]
  Demux/1 -> [usd]
  Demux1/2 -> [isq]
  Demux/2 -> [usq]
  isdq/1 -> Demux1/1
  usdq/1 -> Demux/1
  [usq] -> Add4/2
  K6/1 -> Add4/1
  in_Q_PI/1(Out1) -> Add/1
  Sum23/1 -> in_Q_PI/1(In1)
  [isd] -> Product1/1
  [isq] -> Sum23/2, Scope3/2
  Product1/1 -> K6/1
  Constant4/1 -> Product1/2
  Add4/1 -> Add/2
  Real-Imag to Complex/1 -> Complex to Magnitude-Angle/1
  Complex to Magnitude-Angle/1 -> Magnitude-Angle to Complex/1
  Complex to Real-Imag1/1 -> ucx/1
  Complex to Real-Imag1/2 -> ucy/1
  [usd] -> Scope1/1, control_AC_voltage/1(usd)
  control_AC_voltage/1(isdref) -> Scope7/1, Sum9/1
  [isq] -> Product5/2
  Product5/1 -> Add7/2
  [usd] -> Product5/1
  [isd] -> Product6/2
  Product6/1 -> Add7/1
  [usq] -> Product6/1
  Gain/1 -> Sum/2
  control_AC_voltage1/1(isqref) -> Scope3/1, Sum23/1
  [usq] -> Scope2/1, control_AC_voltage1/1(usq)
  Constant2/1 -> Scope2/2, control_AC_voltage1/2(usqref)
  Add7/1 -> Scope/1, Gain1/1
  Sum2/1 -> Gain/1
  Constant3/1 -> Sum2/2
  Gain1/1 -> Sum2/1
  Sum/1 -> control_AC_voltage/2(usdref)
  Constant1/1 -> Sum/1

== system M10B39_es_V1/Genrators/ES1/output ==
  is_xy : Inport
  Pe : Inport  Port=2
  Brecx : Constant  Value=0
  Brecy : Constant  Value=0
  Bus Creator : BusCreator  Inputs=4
  Constant : Constant
  Constant4 : Constant  Value=P0
  Gain : Gain  Gain=SvscB./SgridB
  Gain1 : Gain  Gain=-1
  Gain2 : Gain  Gain=-1
  Gain6 : Gain
  Grecx : Constant  Value=0
  Grecy : Constant  Value=0
  Mux3 : Mux
  Sum : Sum  Inputs=|++
  Sum1 : Sum  Inputs=|+-
  m : Outport
  isxy : Outport  Port=2
  GBxy : Outport  Port=3
  wires:
  Bus Creator/1 -> m/1
  Gain6/1 -> GBxy/1, Bus Creator/4  "GBxy"
  Mux3/1 -> Gain6/1
  Grecx/1 -> Mux3/1
  Brecx/1 -> Mux3/3
  Grecy/1 -> Mux3/2
  Brecy/1 -> Mux3/4
  Gain1/1 -> isxy/1, Bus Creator/1  "is_xy"
  Gain/1 -> Gain1/1  "is_xy"
  Pe/1 -> Gain2/1  "Pe"
  [WreES1] -> Sum/1  "Pe"
  Constant/1 -> Sum/2
  Sum/1 -> Bus Creator/3  "w"
  is_xy/1 -> Gain/1
  Gain2/1 -> Sum1/1  "Pe"
  Constant4/1 -> Sum1/2
  Sum1/1 -> Bus Creator/2  "Pe"

== system M10B39_es_V1/Genrators/ES1/xy->dq ==
  Ixy : Inport
  Theta : Inport  Port=2
  Complex to Magnitude-Angle : ComplexToMagnitudeAngle
  Complex to Real-Imag : ComplexToRealImag
  Demux1 : Demux  Outputs=2
      settings: DisplayOption=none
  Magnitude-Angle to Complex : MagnitudeAngleToComplex
  Mux : Mux  Inputs=2
  Real-Imag to Complex : RealImagToComplex
  Scope : Scope
  Scope1 : Scope
  Sum1 : Sum  Inputs=|+-  SaturateOnIntegerOverflow=on
  Idq : Outport
  wires:
  Complex to Magnitude-Angle/1 -> Magnitude-Angle to Complex/1
  Theta/1 -> Sum1/2
  Complex to Magnitude-Angle/2 -> Sum1/1, Scope1/1
  Demux1/1 -> Real-Imag to Complex/1
  Complex to Real-Imag/2 -> Mux/2  "Iq"
  Mux/1 -> Idq/1
  Complex to Real-Imag/1 -> Mux/1  "Id"
  Magnitude-Angle to Complex/1 -> Complex to Real-Imag/1
  Sum1/1 -> Magnitude-Angle to Complex/2, Scope/1
  Demux1/2 -> Real-Imag to Complex/2
  Real-Imag to Complex/1 -> Complex to Magnitude-Angle/1
  Ixy/1 -> Demux1/1

== system M10B39_es_V1/Genrators/ES2/ control1 ==
  usdq : Inport
  isdq : Inport  Port=2
  delta : Inport  Port=3
  Enable : EnablePort
  Add : Sum  Inputs=|-+
  Add2 : Sum  Inputs=|-+
  Add3 : Sum
  Add4 : Sum  Inputs=-+
  Add6 : Sum  Inputs=|++
  Add7 : Sum  Inputs=+-
  Complex to Magnitude-Angle : ComplexToMagnitudeAngle
  Complex to Real-Imag1 : ComplexToRealImag
  Constant : Constant
  Constant1 : Constant  Value=usd0
  Constant2 : Constant  Value=0
  Constant3 : Constant  Value=Q0
  Constant4 : Constant
  Demux : Demux  Outputs=2
  Demux1 : Demux  Outputs=2
  Gain : Gain  Gain=0.01
  Gain1 : Gain  Gain=-1
  K5 : Gain  Gain=Lpr  SaturateOnIntegerOverflow=on  OutDataTypeStr=Inherit: Same as input  ParamDataTypeStr=Inherit: Same as input
  K6 : Gain  Gain=Lpr  SaturateOnIntegerOverflow=on  OutDataTypeStr=Inherit: Same as input  ParamDataTypeStr=Inherit: Same as input
  Magnitude-Angle to Complex : MagnitudeAngleToComplex
  Product{1,4..6} (4 alike) : Product  RndMeth=Zero
  Real-Imag to Complex : RealImagToComplex
  Scope{,1..2,7} (4 alike) : Scope
  Sum : Sum  Inputs=|+-
  Sum2 : Sum  Inputs=|+-  SaturateOnIntegerOverflow=on
  Sum23 : Sum  Inputs=|+-  SaturateOnIntegerOverflow=on
  Sum9 : Sum  Inputs=|+-  SaturateOnIntegerOverflow=on
  control_AC_voltage : Subsystem  VariantControl=VSC1q_Variant2
  control_AC_voltage1 : Subsystem  VariantControl=VSC1q_Variant2
  in_D_PI : Subsystem  mask{KP_=KpId_VSC_A, KI_=KiId_VSC_A, Upper_limit=inf, Lower_limit=-inf, Upper_saturation_limit=inf, Lower_saturation_limit=-inf, integrator_init=Md_A_0}
      mask prompts: KP_ "比例系数P"; KI_ "积分系数I"; Upper_limit "限幅上限"; Lower_limit "限幅下限"; Upper_saturation_limit "积分饱和上限"; Lower_saturation_limit "积分饱和下限"; integrator_init "积分初始值"
      mask DialogControl Container4 Prompt: 控制参数
      mask DialogControl Container5 Prompt: 初始值
      mask Display: disp('PI')
  in_Q_PI : Subsystem  mask{KP_=KpIq_VSC_A, KI_=KiIq_VSC_A, Upper_limit=inf, Lower_limit=-inf, Upper_saturation_limit=inf, Lower_saturation_limit=-inf, integrator_init=Mq_A_0}
      mask prompts: KP_ "比例系数P"; KI_ "积分系数I"; Upper_limit "限幅上限"; Lower_limit "限幅下限"; Upper_saturation_limit "积分饱和上限"; Lower_saturation_limit "积分饱和下限"; integrator_init "积分初始值"
      mask DialogControl Container4 Prompt: 控制参数
      mask DialogControl Container5 Prompt: 初始值
      mask Display: disp('PI')
  ucx : Outport
  ucy : Outport  Port=2
  wires:
  Magnitude-Angle to Complex/1 -> Complex to Real-Imag1/1
  Add/1 -> Real-Imag to Complex/2
  Add2/1 -> Real-Imag to Complex/1
  delta/1 -> Add6/2
  Add6/1 -> Magnitude-Angle to Complex/2
  Complex to Magnitude-Angle/2 -> Add6/1
  Sum9/1 -> in_D_PI/1(In1)
  K5/1 -> Add3/1
  [usd] -> Add3/2
  Add3/1 -> Add2/2
  in_D_PI/1(Out1) -> Add2/1
  Constant/1 -> Product4/2
  [isq] -> Product4/1
  [isd] -> Sum9/2
  Product4/1 -> K5/1
  Demux1/1 -> [isd]
  Demux/1 -> [usd]
  Demux1/2 -> [isq]
  Demux/2 -> [usq]
  isdq/1 -> Demux1/1
  usdq/1 -> Demux/1
  [usq] -> Add4/2
  K6/1 -> Add4/1
  in_Q_PI/1(Out1) -> Add/1
  Sum23/1 -> in_Q_PI/1(In1)
  [isd] -> Product1/1
  [isq] -> Sum23/2
  Product1/1 -> K6/1
  Constant4/1 -> Product1/2
  Add4/1 -> Add/2
  Real-Imag to Complex/1 -> Complex to Magnitude-Angle/1
  Complex to Magnitude-Angle/1 -> Magnitude-Angle to Complex/1
  Complex to Real-Imag1/1 -> ucx/1
  Complex to Real-Imag1/2 -> ucy/1
  [usd] -> Scope1/1, control_AC_voltage/1(usd)
  control_AC_voltage/1(isdref) -> Scope7/1, Sum9/1
  [isq] -> Product5/2
  Product5/1 -> Add7/2
  [usd] -> Product5/1
  [isd] -> Product6/2
  Product6/1 -> Add7/1
  [usq] -> Product6/1
  Gain/1 -> Sum/2
  control_AC_voltage1/1(isqref) -> Sum23/1
  [usq] -> Scope2/1, control_AC_voltage1/1(usq)
  Constant2/1 -> control_AC_voltage1/2(usqref)
  Add7/1 -> Scope/1, Gain1/1
  Sum2/1 -> Gain/1
  Constant3/1 -> Sum2/2
  Gain1/1 -> Sum2/1
  Sum/1 -> control_AC_voltage/2(usdref)
  Constant1/1 -> Sum/1

== system M10B39_es_V1/Genrators/ES2/output ==
  is_xy : Inport
  Pe : Inport  Port=2
  Brecx : Constant  Value=0
  Brecy : Constant  Value=0
  Bus Creator : BusCreator  Inputs=4
  Constant : Constant
  Constant4 : Constant  Value=P0
  Gain : Gain  Gain=SvscB./SgridB
  Gain1 : Gain  Gain=-1
  Gain2 : Gain  Gain=-1
  Gain6 : Gain
  Grecx : Constant  Value=0
  Grecy : Constant  Value=0
  Mux3 : Mux
  Sum : Sum  Inputs=|++
  Sum1 : Sum  Inputs=|+-
  m : Outport
  isxy : Outport  Port=2
  GBxy : Outport  Port=3
  wires:
  Bus Creator/1 -> m/1
  Gain6/1 -> GBxy/1, Bus Creator/4  "GBxy"
  Mux3/1 -> Gain6/1
  Grecx/1 -> Mux3/1
  Brecx/1 -> Mux3/3
  Grecy/1 -> Mux3/2
  Brecy/1 -> Mux3/4
  Gain1/1 -> isxy/1, Bus Creator/1  "is_xy"
  Gain/1 -> Gain1/1  "is_xy"
  Pe/1 -> Gain2/1  "Pe"
  [WreES2] -> Sum/1  "Pe"
  Constant/1 -> Sum/2
  Sum/1 -> Bus Creator/3  "w"
  is_xy/1 -> Gain/1
  Gain2/1 -> Sum1/1  "Pe"
  Constant4/1 -> Sum1/2
  Sum1/1 -> Bus Creator/2  "Pe"

== system M10B39_es_V1/Genrators/ES2/xy->dq ==
  Ixy : Inport
  Theta : Inport  Port=2
  Complex to Magnitude-Angle : ComplexToMagnitudeAngle
  Complex to Real-Imag : ComplexToRealImag
  Demux1 : Demux  Outputs=2
      settings: DisplayOption=none
  Magnitude-Angle to Complex : MagnitudeAngleToComplex
  Mux : Mux  Inputs=2
  Real-Imag to Complex : RealImagToComplex
  Scope : Scope
  Scope1 : Scope
  Sum1 : Sum  Inputs=|+-  SaturateOnIntegerOverflow=on
  Idq : Outport
  wires:
  Complex to Magnitude-Angle/1 -> Magnitude-Angle to Complex/1
  Theta/1 -> Sum1/2
  Complex to Magnitude-Angle/2 -> Sum1/1, Scope1/1
  Demux1/1 -> Real-Imag to Complex/1
  Complex to Real-Imag/2 -> Mux/2  "Iq"
  Mux/1 -> Idq/1
  Complex to Real-Imag/1 -> Mux/1  "Id"
  Magnitude-Angle to Complex/1 -> Complex to Real-Imag/1
  Sum1/1 -> Magnitude-Angle to Complex/2, Scope/1
  Demux1/2 -> Real-Imag to Complex/2
  Real-Imag to Complex/1 -> Complex to Magnitude-Angle/1
  Ixy/1 -> Demux1/1

== system M10B39_es_V1/Genrators/ES3/ control1 ==
  usdq : Inport
  isdq : Inport  Port=2
  delta : Inport  Port=3
  Enable : EnablePort
  Add : Sum  Inputs=|-+
  Add2 : Sum  Inputs=|-+
  Add3 : Sum
  Add4 : Sum  Inputs=-+
  Add6 : Sum  Inputs=|++
  Add7 : Sum  Inputs=+-
  Complex to Magnitude-Angle : ComplexToMagnitudeAngle
  Complex to Real-Imag1 : ComplexToRealImag
  Constant : Constant
  Constant1 : Constant  Value=usd0
  Constant2 : Constant  Value=0
  Constant3 : Constant  Value=Q0
  Constant4 : Constant
  Demux : Demux  Outputs=2
  Demux1 : Demux  Outputs=2
  Gain : Gain  Gain=0.01
  Gain1 : Gain  Gain=-1
  K5 : Gain  Gain=Lpr  SaturateOnIntegerOverflow=on  OutDataTypeStr=Inherit: Same as input  ParamDataTypeStr=Inherit: Same as input
  K6 : Gain  Gain=Lpr  SaturateOnIntegerOverflow=on  OutDataTypeStr=Inherit: Same as input  ParamDataTypeStr=Inherit: Same as input
  Magnitude-Angle to Complex : MagnitudeAngleToComplex
  Product{1,4..6} (4 alike) : Product  RndMeth=Zero
  Real-Imag to Complex : RealImagToComplex
  Scope{,1..2,7} (4 alike) : Scope
  Sum : Sum  Inputs=|+-
  Sum2 : Sum  Inputs=|+-  SaturateOnIntegerOverflow=on
  Sum23 : Sum  Inputs=|+-  SaturateOnIntegerOverflow=on
  Sum9 : Sum  Inputs=|+-  SaturateOnIntegerOverflow=on
  control_AC_voltage : Subsystem  VariantControl=VSC1q_Variant2
  control_AC_voltage1 : Subsystem  VariantControl=VSC1q_Variant2
  in_D_PI : Subsystem  mask{KP_=KpId_VSC_A, KI_=KiId_VSC_A, Upper_limit=inf, Lower_limit=-inf, Upper_saturation_limit=inf, Lower_saturation_limit=-inf, integrator_init=Md_A_0}
      mask prompts: KP_ "比例系数P"; KI_ "积分系数I"; Upper_limit "限幅上限"; Lower_limit "限幅下限"; Upper_saturation_limit "积分饱和上限"; Lower_saturation_limit "积分饱和下限"; integrator_init "积分初始值"
      mask DialogControl Container4 Prompt: 控制参数
      mask DialogControl Container5 Prompt: 初始值
      mask Display: disp('PI')
  in_Q_PI : Subsystem  mask{KP_=KpIq_VSC_A, KI_=KiIq_VSC_A, Upper_limit=inf, Lower_limit=-inf, Upper_saturation_limit=inf, Lower_saturation_limit=-inf, integrator_init=Mq_A_0}
      mask prompts: KP_ "比例系数P"; KI_ "积分系数I"; Upper_limit "限幅上限"; Lower_limit "限幅下限"; Upper_saturation_limit "积分饱和上限"; Lower_saturation_limit "积分饱和下限"; integrator_init "积分初始值"
      mask DialogControl Container4 Prompt: 控制参数
      mask DialogControl Container5 Prompt: 初始值
      mask Display: disp('PI')
  ucx : Outport
  ucy : Outport  Port=2
  wires:
  Magnitude-Angle to Complex/1 -> Complex to Real-Imag1/1
  Add/1 -> Real-Imag to Complex/2
  Add2/1 -> Real-Imag to Complex/1
  delta/1 -> Add6/2
  Add6/1 -> Magnitude-Angle to Complex/2
  Complex to Magnitude-Angle/2 -> Add6/1
  Sum9/1 -> in_D_PI/1(In1)
  K5/1 -> Add3/1
  [usd] -> Add3/2
  Add3/1 -> Add2/2
  in_D_PI/1(Out1) -> Add2/1
  Constant/1 -> Product4/2
  [isq] -> Product4/1
  [isd] -> Sum9/2
  Product4/1 -> K5/1
  Demux1/1 -> [isd]
  Demux/1 -> [usd]
  Demux1/2 -> [isq]
  Demux/2 -> [usq]
  isdq/1 -> Demux1/1
  usdq/1 -> Demux/1
  [usq] -> Add4/2
  K6/1 -> Add4/1
  in_Q_PI/1(Out1) -> Add/1
  Sum23/1 -> in_Q_PI/1(In1)
  [isd] -> Product1/1
  [isq] -> Sum23/2
  Product1/1 -> K6/1
  Constant4/1 -> Product1/2
  Add4/1 -> Add/2
  Real-Imag to Complex/1 -> Complex to Magnitude-Angle/1
  Complex to Magnitude-Angle/1 -> Magnitude-Angle to Complex/1
  Complex to Real-Imag1/1 -> ucx/1
  Complex to Real-Imag1/2 -> ucy/1
  [usd] -> Scope1/1, control_AC_voltage/1(usd)
  control_AC_voltage/1(isdref) -> Scope7/1, Sum9/1
  [isq] -> Product5/2
  Product5/1 -> Add7/2
  [usd] -> Product5/1
  [isd] -> Product6/2
  Product6/1 -> Add7/1
  [usq] -> Product6/1
  Gain/1 -> Sum/2
  control_AC_voltage1/1(isqref) -> Sum23/1
  [usq] -> Scope2/1, control_AC_voltage1/1(usq)
  Constant2/1 -> control_AC_voltage1/2(usqref)
  Add7/1 -> Scope/1, Gain1/1
  Sum2/1 -> Gain/1
  Constant3/1 -> Sum2/2
  Gain1/1 -> Sum2/1
  Sum/1 -> control_AC_voltage/2(usdref)
  Constant1/1 -> Sum/1

== system M10B39_es_V1/Genrators/ES3/in_D_PI ==
  In1 : Inport
  Ki : Gain  Gain=KI_  SaturateOnIntegerOverflow=on  OutDataTypeStr=Inherit: Same as input  ParamDataTypeStr=Inherit: Same as input
  Kp : Gain  Gain=KP_  SaturateOnIntegerOverflow=on  OutDataTypeStr=Inherit: Same as input  ParamDataTypeStr=Inherit: Same as input
  Saturation2 : Saturate  UpperLimit=Upper_limit  LowerLimit=Lower_limit
  Sum12 : Sum  SaturateOnIntegerOverflow=on
  integrator : Integrator  InitialCondition=integrator_init  LimitOutput=on  UpperSaturationLimit=Upper_saturation_limit  LowerSaturationLimit=Lower_saturation_limit
  Out1 : Outport
  wires:
  In1/1 -> Ki/1, Kp/1
  Kp/1 -> Sum12/2
  Ki/1 -> integrator/1
  integrator/1 -> Sum12/1
  Saturation2/1 -> Out1/1
  Sum12/1 -> Saturation2/1

== system M10B39_es_V1/Genrators/ES3/output ==
  is_xy : Inport
  Pe : Inport  Port=2
  Brecx : Constant  Value=0
  Brecy : Constant  Value=0
  Bus Creator : BusCreator  Inputs=4
  Constant : Constant
  Gain : Gain  Gain=SvscB./SgridB
  Gain1 : Gain  Gain=-1
  Gain2 : Gain  Gain=-1
  Gain6 : Gain
  Grecx : Constant  Value=0
  Grecy : Constant  Value=0
  Mux3 : Mux
  Sum : Sum  Inputs=|++
  m : Outport
  isxy : Outport  Port=2
  GBxy : Outport  Port=3
  wires:
  Bus Creator/1 -> m/1
  Gain6/1 -> GBxy/1, Bus Creator/4  "GBxy"
  Mux3/1 -> Gain6/1
  Grecx/1 -> Mux3/1
  Brecx/1 -> Mux3/3
  Grecy/1 -> Mux3/2
  Brecy/1 -> Mux3/4
  Gain1/1 -> isxy/1, Bus Creator/1  "is_xy"
  Gain2/1 -> Bus Creator/2  "Pe"
  Gain/1 -> Gain1/1  "is_xy"
  Pe/1 -> Gain2/1  "Pe"
  Constant/1 -> Sum/2
  [WreES3] -> Sum/1  "Pe"
  Sum/1 -> Bus Creator/3  "w"
  is_xy/1 -> Gain/1

== system M10B39_es_V1/Genrators/ES3/xy->dq ==
  Ixy : Inport
  Theta : Inport  Port=2
  Complex to Magnitude-Angle : ComplexToMagnitudeAngle
  Complex to Real-Imag : ComplexToRealImag
  Demux1 : Demux  Outputs=2
      settings: DisplayOption=none
  Magnitude-Angle to Complex : MagnitudeAngleToComplex
  Mux : Mux  Inputs=2
  Real-Imag to Complex : RealImagToComplex
  Scope : Scope
  Scope1 : Scope
  Sum1 : Sum  Inputs=|+-  SaturateOnIntegerOverflow=on
  Idq : Outport
  wires:
  Complex to Magnitude-Angle/1 -> Magnitude-Angle to Complex/1
  Theta/1 -> Sum1/2
  Complex to Magnitude-Angle/2 -> Sum1/1, Scope1/1
  Demux1/1 -> Real-Imag to Complex/1
  Complex to Real-Imag/2 -> Mux/2  "Iq"
  Mux/1 -> Idq/1
  Complex to Real-Imag/1 -> Mux/1  "Id"
  Magnitude-Angle to Complex/1 -> Complex to Real-Imag/1
  Sum1/1 -> Magnitude-Angle to Complex/2, Scope/1
  Demux1/2 -> Real-Imag to Complex/2
  Real-Imag to Complex/1 -> Complex to Magnitude-Angle/1
  Ixy/1 -> Demux1/1

== system M10B39_es_V1/Genrators/Generator1/Excitation System ST1A1 ==
  note: Ef
  Upss : Inport
  Trip : Inport  Port=2
  Vg : Inport  Port=3
  Constant1 : Constant  Value=0
  Ef1 : Integrator  InitialCondition=Ef10
  K : Gain  Gain=1/Tb  SaturateOnIntegerOverflow=on  OutDataTypeStr=Inherit: Same as input  ParamDataTypeStr=Inherit: Same as input
  KA : Gain  Gain=Ka  SaturateOnIntegerOverflow=on  OutDataTypeStr=Inherit: Same as input  ParamDataTypeStr=Inherit: Same as input
  KA1 : Gain  Gain=Tc/Tb  SaturateOnIntegerOverflow=on  OutDataTypeStr=Inherit: Same as input  ParamDataTypeStr=Inherit: Same as input
  KA2 : Gain  Gain=(1/Tb)*(1-Tc/Tb)  SaturateOnIntegerOverflow=on  OutDataTypeStr=Inherit: Same as input  ParamDataTypeStr=Inherit: Same as input
  Saturation : Saturate  UpperLimit=Efmax  LowerLimit=Efmin
  Sum : Sum  Inputs=|++  SaturateOnIntegerOverflow=on
  Sum1 : Sum  Inputs=|+-  SaturateOnIntegerOverflow=on
  Sum4 : Sum  Inputs=|+-+  SaturateOnIntegerOverflow=on
  Switch2 : Switch  Criteria=u2 ~= 0  Threshold=0.5  InputSameDT=off
  Switch3 : Switch  Criteria=u2 ~= 0  Threshold=0.5  InputSameDT=off
  Vref : Constant  Value=Vref
  Ef : Outport
  wires:
  Trip/1 -> Switch3/2, Switch2/2
  Constant1/1 -> Switch3/1, Switch2/1
  Switch3/1 -> KA2/1, K/1
  Ef1/1 -> Switch3/3
  Switch2/1 -> Ef1/1
  Sum1/1 -> Switch2/3
  KA/1 -> KA1/1, Sum1/1
  Upss/1 -> Sum4/3
  Saturation/1 -> Ef/1
  Vg/1 -> Sum4/2
  Sum4/1 -> KA/1
  Vref/1 -> Sum4/1
  Sum/1 -> Saturation/1
  K/1 -> Sum1/2
  KA1/1 -> Sum/2
  KA2/1 -> Sum/1

== system M10B39_es_V1/Genrators/Generator1/Governor ==
  w : Inport
  Trip : Inport  Port=2
  CT : Constant  Value=0
  Constant : Constant  Value=0
  Gain : Gain  Gain=a_G  SaturateOnIntegerOverflow=on  OutDataTypeStr=Inherit: Same as input  ParamDataTypeStr=Inherit: Same as input
  Saturation : Saturate  UpperLimit=dPmax  LowerLimit=dPmin
  Sum1 : Sum  Inputs=|++  SaturateOnIntegerOverflow=on
  Sum3 : Sum  Inputs=|+-  SaturateOnIntegerOverflow=on
  Switch : Switch  Threshold=0.5  InputSameDT=off
  Switch1 : Switch  Criteria=u2 ~= 0  Threshold=0.5  InputSameDT=off
  Transfer Fcn1 : TransferFcn  Numerator=[b_G]  Denominator=[Tg_G 1]
  w0 : Gain  Gain=wB  SaturateOnIntegerOverflow=on  OutDataTypeStr=Inherit: Same as input  ParamDataTypeStr=Inherit: Same as input
  w1 : Constant  Value=S_Gov
  wref : Constant
  dPm : Outport
  wires:
  Gain/1 -> Sum1/1
  w1/1 -> Switch/2
  CT/1 -> Switch/3
  Sum3/1 -> w0/1
  Sum1/1 -> Saturation/1
  Saturation/1 -> Switch/1
  wref/1 -> Sum3/1
  w0/1 -> Gain/1, Transfer Fcn1/1
  Transfer Fcn1/1 -> Sum1/2
  w/1 -> Sum3/2
  Constant/1 -> Switch1/1
  Switch/1 -> Switch1/3
  Trip/1 -> Switch1/2
  Switch1/1 -> dPm/1

== system M10B39_es_V1/Genrators/Generator1/Machine Equations  ==
  note: Iqg
  note: Idg
  note: 接口
  delta : Inport
  Vgxy : Inport  Port=2
  Ef : Inport  Port=3
  Trip : Inport  Port=4
  Demux : Demux  Outputs=2
  Demux1 : Demux  Outputs=2
  Fcn1 : Fcn  Expr=u(1)*u(3)+u(2)*u(4)
  Fcn2 : Fcn  Expr=(u(3)-u(2))/Xd1
  Fcn3 : Fcn  Expr=(u(1)-u(4))/Xq1
  Fcn4 : Fcn  Expr=u(2)*u(3)-u(1)*u(4)
  Fcn6 : Fcn  Expr=sqrt(u(1)^2+u(2)^2)
  Interface : Subsystem
  Mux1 : Mux  Inputs=2
  Mux2 : Mux  Inputs=2
  Mux3 : Mux  Inputs=2
  Qe : Scope
  Scope{,1..3} (4 alike) : Scope
  Transient Equations : Subsystem
  Pe : Outport
  Igxy1 : Outport  Port=2
  GBxy : Outport  Port=3
  Vg : Outport  Port=4
  wires:
  Trip/1 -> Transient Equations/3(Trip)
  Demux1/2 -> Scope3/1
  Demux/2 -> Scope2/1
  Demux1/1 -> Scope/1
  Demux/1 -> Scope1/1
  Transient Equations/1(Eqd') -> Interface/3(Eqd''), Mux1/2
  Interface/3(GBxy) -> GBxy/1
  Interface/2(Igxy1) -> Igxy1/1
  Vgxy/1 -> Interface/2(Vgxy)
  delta/1 -> Interface/1(delta)
  Fcn4/1 -> Qe/1
  Fcn6/1 -> Vg/1
  Fcn1/1 -> Pe/1
  Ef/1 -> Transient Equations/2(Ef)
  Mux2/1 -> Fcn4/1, Fcn1/1
  Mux1/1 -> Fcn3/1, Fcn2/1
  Interface/1(Vdqg) -> Mux1/1, Fcn6/1, Mux2/1, Demux/1
  Mux3/1 -> Mux2/2, Demux1/1, Transient Equations/1(Idqg)
  Fcn2/1 -> Mux3/1
  Fcn3/1 -> Mux3/2

== system M10B39_es_V1/Genrators/Generator1/Mechanical DE ==
  Pe : Inport
  dPm : Inport  Port=2
  Trip : Inport  Port=3
  Constant1 : Constant  Value=0
  Constant2 : Constant  Value=0
  Gain : Gain  Gain=wB  SaturateOnIntegerOverflow=on  OutDataTypeStr=Inherit: Same as input  ParamDataTypeStr=Inherit: Same as input
  Gain1 : Gain  Gain=1/H  SaturateOnIntegerOverflow=on  OutDataTypeStr=Inherit: Same as input  ParamDataTypeStr=Inherit: Same as input
  Gain2 : Gain  Gain=D  SaturateOnIntegerOverflow=on  OutDataTypeStr=Inherit: Same as input  ParamDataTypeStr=Inherit: Same as input
  Gain5 : Gain  Gain=180/pi  SaturateOnIntegerOverflow=on  OutDataTypeStr=Inherit: Same as input  ParamDataTypeStr=Inherit: Same as input
  Int1 : Integrator  InitialCondition=delta0
  Int2 : Integrator  InitialCondition=w0
  Pm : Constant  Value=Pm0
  Scope2 : Scope
  Scope4 : Scope
  Scope8 : Scope
  Sum2 : Sum  Inputs=-+-+  SaturateOnIntegerOverflow=on
  Sum3 : Sum  Inputs=|+-  SaturateOnIntegerOverflow=on
  Switch{1..4} (4 alike) : Switch  Criteria=u2 ~= 0  Threshold=0.5  InputSameDT=off
  w0 : Constant
  delta : Outport
  w : Outport  Port=2
  wires:
  [Trip] -> Switch3/2, Switch2/2
  Constant1/1 -> Switch3/1, Switch2/1
  Switch3/1 -> Scope4/1, Sum3/1, w/1
  Int2/1 -> Switch3/3
  Switch2/1 -> Int2/1
  Gain1/1 -> Switch2/3
  Trip/1 -> [Trip]
  [Trip] -> Switch1/2, Switch4/2
  Constant2/1 -> Switch4/1, Switch1/1
  Switch4/1 -> delta/1, Scope2/1, Gain5/1
  Int1/1 -> Switch4/3
  Switch1/1 -> Int1/1
  Gain/1 -> Switch1/3
  Gain5/1 -> Scope8/1
  w0/1 -> Sum3/2
  Sum3/1 -> Gain2/1, Gain/1
  Pm/1 -> Sum2/2
  Gain2/1 -> Sum2/1
  Sum2/1 -> Gain1/1
  Pe/1 -> Sum2/3
  dPm/1 -> Sum2/4

== system M10B39_es_V1/Genrators/Generator1/Output ==
  Igxy1in : Inport
  GBxyin : Inport  Port=2
  deltain : Inport  Port=3
  Pein : Inport  Port=4
  fin : Inport  Port=5
  Vg : Inport  Port=6
  Bus Creator : BusCreator  Inputs=6
  m : Outport
  Igxy1 : Outport  Port=2
  GBxy : Outport  Port=3
  wires:
  Vg/1 -> Bus Creator/6  "Vg"
  fin/1 -> Bus Creator/5  "f"
  Pein/1 -> Bus Creator/4  "Pe"
  deltain/1 -> Bus Creator/3  "delta"
  GBxyin/1 -> Bus Creator/2, GBxy/1  "GBxy"
  Igxy1in/1 -> Bus Creator/1, Igxy1/1  "Igxy1"
  Bus Creator/1 -> m/1
